simulink model "PiekarekLab6_si"  (R2022b)
settings: Solver=VariableStepAuto  StartTime=0.0  StopTime=czas  MaxStep=5  RelTol=1e-3
values from neighbouring files (symbols this model uses):
  cpp = 1000    [PiekarekLabNr6.m]
  Cvp = cpp*rop*Vp    (= 24000)    [PiekarekLabNr6.m]
  Cvv = cpp*rop*Vw    (= 12000)    [PiekarekLabNr6.m]
  czas_skok = 300    [PiekarekLabNr6.m]
  dFp = 0    [PiekarekLabNr6.m]
  dTzew = 0    [PiekarekLabNr6.m]
  Fp0 = fPN*25    (= 0.0231481481481)    [PiekarekLabNr6.m]
  K1 = 2*Kd    (= 260.096618357)    [PiekarekLabNr6.m]
  Kd = (PgN-cpp*rop*fPN*(TwewN-TzewN))/(2*(TwewN-TzewN) +7*(TwewN-TpN))    (= 130.048309179)    [PiekarekLabNr6.m]
  Kp = (Kd*(TpN-TzewN))/(TwewN-TpN)    (= 910.338164251)    [PiekarekLabNr6.m]
  Kp1 = (0.9*T)/(k*T0)    (= 2100)    [PiekarekLabNr6.m]
  Pg0 = PgN    (= 15000)    [PiekarekLabNr6.m]
  rop = 1.2    [PiekarekLabNr6.m]
  Ti = 3.33*T0    (= 66.6)    [PiekarekLabNr6.m]
  Tp0 = (Kp*Twew0+Kd*Tzew0)/(Kp+Kd)    (= 15)    [PiekarekLabNr6.m]
  Twew0 = Tzew0+(Pg0/(K1+(cpp*rop*Fp0)+(Kp*Kd)/(Kp+Kd)))    (= 20)    [PiekarekLabNr6.m]
  Tzad = Tzad0+dTzad    (= 30)    [PiekarekLabNr6.m]
  Tzad0 = Tp0+10    (= 25)    [PiekarekLabNr6.m]
  Tzew0 = TzewN+3    (= -17)    [PiekarekLabNr6.m]
settings Model: Creator=Lenovo  LastModifiedBy=Lenovo

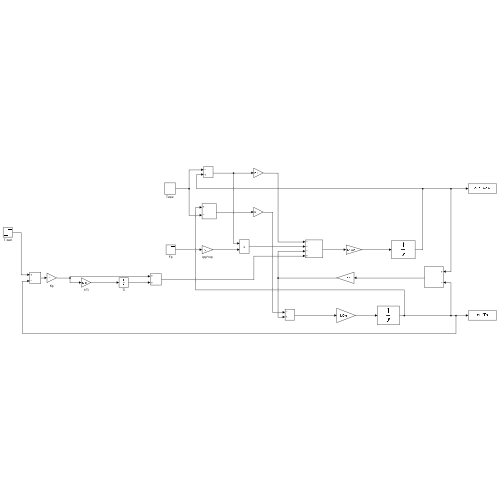
[thumbnail: Simulink's stored preview of the top-level diagram]
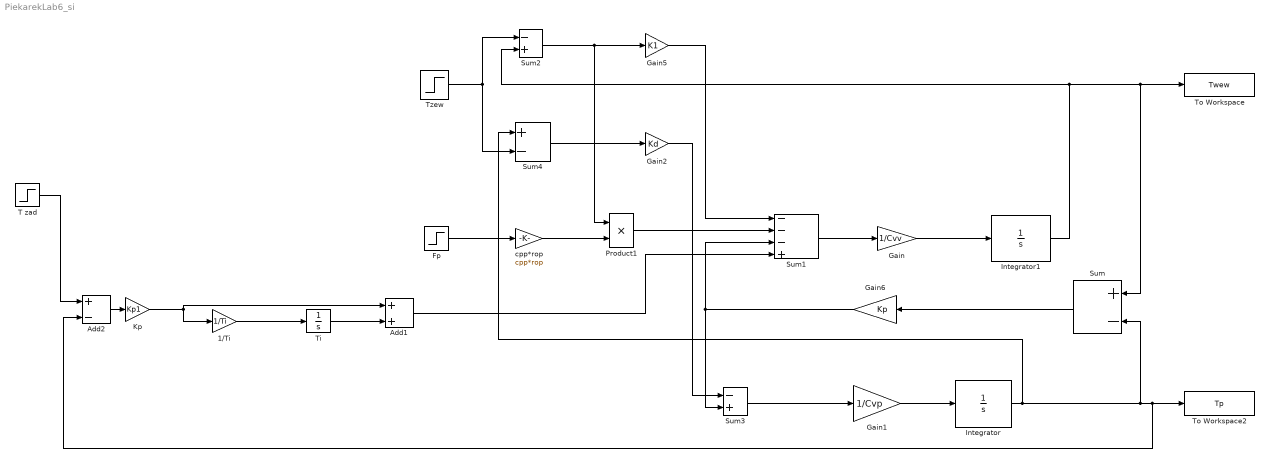
== system PiekarekLab6_si ==
  1/Ti : Gain  Gain=1/Ti
  Add1 : Sum
  Add2 : Sum  Inputs=+-
  Fp : Step  Time=czas_skok  Before=Fp0  After=Fp0+dFp  SampleTime=0
  Gain : Gain  Gain=1/Cvv
  Gain1 : Gain  Gain=1/Cvp
  Gain2 : Gain  Gain=Kd
  Gain5 : Gain  Gain=K1
  Gain6 : Gain  Gain=Kp
  Integrator : Integrator  InitialCondition=Tp0
  Integrator1 : Integrator  InitialCondition=Twew0
  Kp : Gain  Gain=Kp1
  Product1 : Product
  Sum : Sum  Inputs=+-
  Sum1 : Sum  Inputs=---+
  Sum2 : Sum  Inputs=-+
  Sum3 : Sum  Inputs=-+
  Sum4 : Sum  Inputs=+-
  T zad : Step  Time=czas_skok  Before=Tzad0  After=Tzad  SampleTime=0
  Ti : Integrator  InitialCondition=Pg0
  To Workspace : ToWorkspace  VariableName=Twew  SampleTime=-1
  To Workspace2 : ToWorkspace  VariableName=Tp  SampleTime=-1
  Tzew : Step  Time=czas_skok  Before=Tzew0  After=Tzew0+dTzew  SampleTime=0
  cpp*rop : Gain  Gain=cpp*rop
  wires:
  Gain2/1 -> Sum3/1
  Gain5/1 -> Sum1/1
  Sum2/1 -> Product1/1, Gain5/1
  Sum1/1 -> Gain/1
  Sum3/1 -> Gain1/1
  Gain6/1 -> Sum1/3, Sum3/2
  Integrator1/1 -> Sum2/2, To Workspace/1, Sum/1
  Sum/1 -> Gain6/1
  Product1/1 -> Sum1/2
  Fp/1 -> cpp*rop/1
  Sum4/1 -> Gain2/1
  Tzew/1 -> Sum4/2, Sum2/1
  Gain/1 -> Integrator1/1
  Integrator/1 -> Sum4/1, Sum/2, Add2/2, To Workspace2/1
  cpp*rop/1 -> Product1/2
  Gain1/1 -> Integrator/1
  Add1/1 -> Sum1/4
  T zad/1 -> Add2/1
  Ti/1 -> Add1/2
  Add2/1 -> Kp/1
  1/Ti/1 -> Ti/1
  Kp/1 -> 1/Ti/1, Add1/1
